simulink model "sdl_hybrid_series"  (R2019b)
settings: Solver=VariableStepAuto  StartTime=0.0  StopTime=20  RelTol=1e-3  AbsTol=1e-3  EnableMultiTasking=on
model workspace (MATLAB code in the model file):
  | v0                 = 15; % Initial vehicle speed
  | wheel_radius = 0.3; % Wheel radius
  | k                   = 1e-2; % Motor losses (W/(N*M)^2)
  | t_torque        = 0.02; % Electric motor time constant
  | rpm0             = 2000; % Engine initial speed demand
libraries: fl_lib x31, fl_ps_legacy_lib x25, nesl_utility x13, sdl_lib x4
(part 2 of 2)

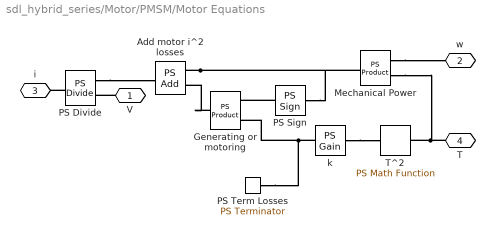
== system sdl_hybrid_series/Motor/PMSM/Motor Equations ==
  Add motor i^2 losses : fl_ps_legacy_lib/Legacy Physical Signals/Functions/PS Add
      settings: SourceProductName=Simscape  SourceProductBaseCode=SS  InternalSimscapePortConfiguration="{\"Bottom\":[],\"Left\":[{\"id\":\"I1\",\"label\":\"\",\"type\":\"input\"},{\"id\":\"I2\",\"label\":\"\",\"type\":\"input\"}],\"Right\":[{\"id\":\"O\",\"label\":\"\",\"type\":\"output\"}],\"Top\":[]}"
  Generating or motoring : fl_ps_legacy_lib/Legacy Physical Signals/Functions/PS Product
      settings: SourceProductName=Simscape  SourceProductBaseCode=SS
  Mechanical Power : fl_ps_legacy_lib/Legacy Physical Signals/Functions/PS Product
      settings: SourceProductName=Simscape  SourceProductBaseCode=SS
  PS Divide : fl_ps_legacy_lib/Legacy Physical Signals/Functions/PS Divide
      settings: SourceProductName=Simscape  SourceProductBaseCode=SS  InternalSimscapePortConfiguration="{\"Bottom\":[],\"Left\":[{\"id\":\"I1\",\"label\":\"\",\"type\":\"input\"},{\"id\":\"I2\",\"label\":\"\",\"type\":\"input\"}],\"Right\":[{\"id\":\"O\",\"label\":\"\",\"type\":\"output\"}],\"Top\":[]}"
  PS Sign : fl_ps_legacy_lib/Legacy Physical Signals/Nonlinear Operators/PS Sign
      settings: SourceProductName=Simscape  SourceProductBaseCode=SS  InternalSimscapePortConfiguration="{\"Bottom\":[],\"Left\":[{\"id\":\"I\",\"label\":\"\",\"type\":\"input\"}],\"Right\":[{\"id\":\"O\",\"label\":\"\",\"type\":\"output\"}],\"Top\":[]}"
  PS Term Losses : fl_lib/Physical Signals/Sinks/PS Terminator
      settings: SourceProductName=Simscape
  T^2 : fl_ps_legacy_lib/Legacy Physical Signals/Functions/PS Math Function  fcn_choice=7
      settings: SourceProductName=Simscape  SourceProductBaseCode=SS  InternalSimscapePortConfiguration="{\"Bottom\":[],\"Left\":[{\"id\":\"I\",\"label\":\"\",\"type\":\"input\"}],\"Right\":[{\"id\":\"O\",\"label\":\"\",\"type\":\"output\"}],\"Top\":[]}"
  k : fl_ps_legacy_lib/Legacy Physical Signals/Functions/PS Gain  gain=k
      settings: SourceProductName=Simscape
  V : PMIOPort  Side=Left
  w : PMIOPort  Port=2  Side=Right
  i : PMIOPort  Port=3  Side=Left
  T : PMIOPort  Port=4  Side=Right
  connections:
  k/LConn1 -- T^2/RConn1
  Mechanical Power/LConn2 -- T/RConn1 -- T^2/LConn1
  k/RConn1 -- Generating or motoring/LConn2 -- PS Term Losses/LConn1
  Mechanical Power/LConn1 -- w/RConn1
  PS Divide/LConn1 -- Add motor i^2 losses/RConn1
  Generating or motoring/RConn1 -- Add motor i^2 losses/LConn2
  PS Sign/RConn1 -- Generating or motoring/LConn1
  Add motor i^2 losses/LConn1 -- PS Sign/LConn1 -- Mechanical Power/RConn1
  PS Divide/RConn1 -- i/RConn1
  V/RConn1 -- PS Divide/LConn2

== system sdl_hybrid_series/Motor/PMSM/Speed Torque Interface ==
  Motion Sensor : fl_lib/Mechanical/Mechanical Sensors/Ideal Rotational Motion Sensor  offset=0 rad
  Torque Source : fl_lib/Mechanical/Mechanical Sources/Ideal Torque Source
  w : PMIOPort  Side=Left
  R : PMIOPort  Port=2  Side=Left
  T : PMIOPort  Port=3  Side=Right
  C : PMIOPort  Port=4  Side=Right
  connections:
  Motion Sensor/RConn1 -- Torque Source/RConn2 -- C/RConn1
  Torque Source/LConn1 -- R/RConn1 -- Motion Sensor/LConn1
  w/RConn1 -- Motion Sensor/RConn2
  T/RConn1 -- Torque Source/RConn1

== system sdl_hybrid_series/Motor/PMSM/Voltage Current Interface ==
  Controlled Current Source : fl_lib/Electrical/Electrical Sources/Controlled Current Source
  Voltage Sensor : fl_lib/Electrical/Electrical Sensors/Voltage Sensor
  + : PMIOPort  Side=Left
  - : PMIOPort  Port=2  Side=Right
  i : PMIOPort  Port=3  Side=Right
  V : PMIOPort  Port=4  Side=Left
  connections:
  Controlled Current Source/RConn2 -- Voltage Sensor/LConn1 -- +/RConn1
  Voltage Sensor/RConn1 -- V/RConn1
  i/RConn1 -- Controlled Current Source/RConn1
  -/RConn1 -- Controlled Current Source/LConn1 -- Voltage Sensor/RConn2
